simulink model "dp_reference_model"  (R2020a)
settings: Solver=FixedStepAuto  StartTime=0.0  StopTime=10.0  FixedStep=0.01  RelTol=1e-3
PreLoadFcn:
  | load("interfaces.mat");
undefined symbols (not defined in the file or in its folder): east, north, yaw
settings Model: Creator=thomas.evang  LastModifiedBy=thomas.evang
settings SFSimCC: CustomCodeUndefinedFunction=UseInterfaceOnly
settings RTWCC: Description=Generic Real-Time Target  RetainRTWFile=on

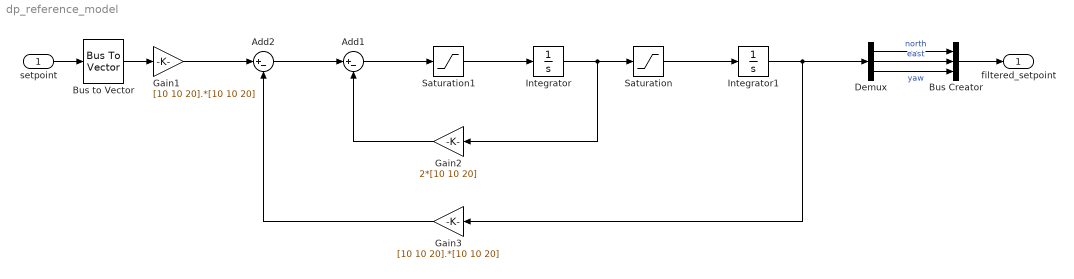
== system dp_reference_model ==
  setpoint : Inport  OutDataTypeStr=Bus: position_3dof
  Add1 : Sum  Inputs=|+-
  Add2 : Sum  Inputs=|+-
  Bus Creator : BusCreator  Inputs=north,east,yaw  OutDataTypeStr=Bus: position_3dof
  Bus to Vector : BusToVector
  Demux : Demux  Outputs=3
  Gain1 : Gain  Gain=[10 10 20].*[10 10 20]
  Gain2 : Gain  Gain=2*[10 10 20]
  Gain3 : Gain  Gain=[10 10 20].*[10 10 20]
  Integrator : Integrator  InitialCondition=0*1*[1 1 1]  ZeroCross=off
  Integrator1 : Integrator  InitialCondition=0*1*[1 1 1]  ZeroCross=off
  Saturation : Saturate  UpperLimit=1*[1 1 pi/18/6]  LowerLimit=-1*[1 1 pi/18/6]  ZeroCross=off
  Saturation1 : Saturate  UpperLimit=1*[5 5 1]  LowerLimit=-1*[5 5 1]  ZeroCross=off
  filtered_setpoint : Outport  OutDataTypeStr=Bus: position_3dof  VectorParamsAs1DForOutWhenUnconnected=off
  wires:
  Saturation/1 -> Integrator1/1
  Add1/1 -> Saturation1/1
  Integrator/1 -> Gain2/1, Saturation/1
  Gain1/1 -> Add2/1
  Gain2/1 -> Add1/2
  Add2/1 -> Add1/1
  Gain3/1 -> Add2/2
  setpoint/1 -> Bus to Vector/1
  Saturation1/1 -> Integrator/1
  Integrator1/1 -> Gain3/1, Demux/1
  Bus to Vector/1 -> Gain1/1
  Demux/1 -> Bus Creator/1  "north"
  Demux/2 -> Bus Creator/2  "east"
  Demux/3 -> Bus Creator/3  "yaw"
  Bus Creator/1 -> filtered_setpoint/1
